simulink model "TrajectoryTracking_2015b_00"  (R2016a)
settings: Solver=ode45  SolverMode=SingleTasking  StartTime=0.0  StopTime=200  RelTol=1e-3
values from neighbouring files (symbols this model uses):
  B_input = B_T    [ErrorDynamicsControllerDesign.m]
undefined symbols (not defined in the file or in its folder): angular_velocity_pitch_1, angular_velocity_pitch_2, angular_velocity_pitch_3, angular_velocity_pitch_4, angular_velocity_pitch_5, angular_velocity_pitch_6, angular_velocity_roll_1, angular_velocity_roll_2, angular_velocity_roll_3, angular_velocity_roll_4, angular_velocity_roll_5, angular_velocity_roll_6, angular_velocity_roll_7, angular_velocity_yaw_1, angular_velocity_yaw_2, angular_velocity_yaw_3, angular_velocity_yaw_4, angular_velocity_yaw_5, angular_velocity_yaw_6, angular_velocity_yaw_7, K1, K2, K3, K4, K5, K6, K7, linear_velocity_x_1, linear_velocity_x_2, linear_velocity_x_3, linear_velocity_x_4, linear_velocity_x_5, linear_velocity_x_6, linear_velocity_x_7, linear_velocity_y_1, linear_velocity_y_2, linear_velocity_y_3, linear_velocity_y_4, linear_velocity_y_5, linear_velocity_y_6, linear_velocity_y_7, linear_velocity_z_1, linear_velocity_z_2, linear_velocity_z_3, linear_velocity_z_4, linear_velocity_z_5, linear_velocity_z_6, linear_velocity_z_7, pitch_angle_1, pitch_angle_2, pitch_angle_3, pitch_angle_4, pitch_angle_5, pitch_angle_6, pitch_angle_7, roll_angle_1, roll_angle_2, roll_angle_3, roll_angle_4, roll_angle_5 ... (+59)
undefined symbols (not defined in the file): b_T1_optimized, b_T2_optimized, b_T3_optimized, b_T4_optimized, b_T5_optimized, b_T6_optimized, d_T1_optimized, d_T2_optimized, d_T3_optimized, d_T4_optimized, d_T5_optimized, d_T6_optimized, r_T1_optimized, r_T2_optimized, r_T3_optimized, r_T4_optimized, r_T5_optimized, r_T6_optimized
libraries: aerolibtransform2 x1, aerolib6dofsys x1
(part 1 of 2)
settings Model: Creator=yongyu  LastModifiedBy=ychen
settings DebuggingCC: SFUnexpectedBacktrackingDiag=error  SFNoUnconditionalDefaultTransitionDiag=error
settings GRTTargetCC: TargetLangStandard=C99 (ISO)  GeneratePreprocessorConditionals=Use local settings
settings ConfigComp: CovMetricSettings=dwe  CovHtmlReporting=off  CovSaveCumulativeToWorkspaceVar=off  CovSaveSingleToWorkspaceVar=off  CovModelRefEnable=Off  CovExternalEMLEnable=on

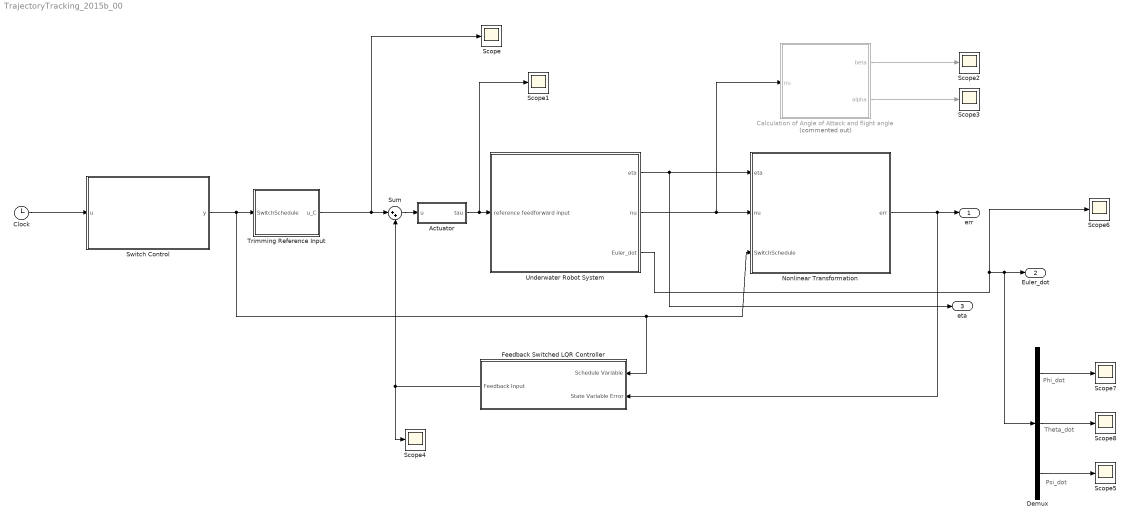
== system TrajectoryTracking_2015b_00 ==
  note: Theta_dot
  note: Phi_dot
  note: Psi_dot
  Actuator : Subsystem
  Calculation of Angle of Attack and flight angle : Subsystem  Commented=on
  Clock : Clock
  Demux : Demux  Outputs=3
  Feedback Switched LQR Controller : Subsystem
  Nonlinear Transformation : Subsystem
  Scope{,1..8} (9 alike) : Scope
  Sum : Sum  Inputs=|++
  Switch Control : MATLAB Function  TreatAsAtomicUnit=on
  "Trimming Reference Input " : Subsystem
  Underwater Robot System : Subsystem
  err : Outport
  Euler_dot : Outport  Port=2
  eta : Outport  Port=3
  wires:
  Nonlinear Transformation/1(err) -> err/1, Feedback Switched LQR Controller/2(State Variable Error)
  Calculation of Angle of Attack and flight angle/2(alpha) -> Scope3/1
  Calculation of Angle of Attack and flight angle/1(beta) -> Scope2/1
  "Trimming Reference Input "/1(u_C) -> Scope/1, Sum/1
  Underwater Robot System/1(eta) -> eta/1, Nonlinear Transformation/1(eta)
  Underwater Robot System/2(nu) -> Calculation of Angle of Attack and flight angle/1(nu), Nonlinear Transformation/2(nu)
  Underwater Robot System/3(Euler_dot) -> Scope6/1, Demux/1, Euler_dot/1
  Clock/1 -> Switch Control/1(u)
  Demux/3 -> Scope5/1
  Switch Control/1(y) -> Feedback Switched LQR Controller/1(Schedule Variable), Nonlinear Transformation/3(SwitchSchedule), "Trimming Reference Input "/1(SwitchSchedule)
  Demux/1 -> Scope7/1
  Demux/2 -> Scope8/1
  Sum/1 -> Actuator/1(u)
  Actuator/1(tau) -> Scope1/1, Underwater Robot System/1("reference feedforward input ")
  Feedback Switched LQR Controller/1(Feedback Input) -> Sum/2, Scope4/1

== system TrajectoryTracking_2015b_00/Actuator ==
  u : Inport
  Add : Sum  Inputs=++++++
  Demux : Demux  Outputs=6
  Saturation : Saturate  UpperLimit=[40 40 40 40 40 40]  LowerLimit=[-35 -35 -35 -35 -35 -35]
  Scope{1..6} (6 alike) : Scope
  Thruster Model1 : Subsystem  mask{d_T=d_T1_optimized, b_T=b_T1_optimized, r_T=r_T1_optimized, lambda_T=veh.lambda1}
      mask DialogControl DescTextVar Prompt: Model of Thruster
  Thruster Model2 : Subsystem  mask{d_T=d_T2_optimized, b_T=b_T2_optimized, r_T=r_T2_optimized, lambda_T=veh.lambda2}
      mask DialogControl DescTextVar Prompt: Model of Thruster
  Thruster Model3 : Subsystem  mask{d_T=d_T3_optimized, b_T=b_T3_optimized, r_T=r_T3_optimized, lambda_T=veh.lambda3}
      mask DialogControl DescTextVar Prompt: Model of Thruster
  Thruster Model4 : Subsystem  mask{d_T=d_T4_optimized, b_T=b_T4_optimized, r_T=r_T4_optimized, lambda_T=veh.lambda4}
      mask DialogControl DescTextVar Prompt: Model of Thruster
  Thruster Model5 : Subsystem  mask{d_T=d_T5_optimized, b_T=b_T5_optimized, r_T=r_T5_optimized, lambda_T=veh.lambda5}
      mask DialogControl DescTextVar Prompt: Model of Thruster
  Thruster Model6 : Subsystem  mask{d_T=d_T6_optimized, b_T=b_T6_optimized, r_T=r_T6_optimized, lambda_T=veh.lambda6}
      mask DialogControl DescTextVar Prompt: Model of Thruster
  tau : Outport
  wires:
  Thruster Model5/1(tau) -> Add/5
  Thruster Model3/1(tau) -> Add/3
  Thruster Model4/1(tau) -> Add/4
  Thruster Model2/1(tau) -> Add/2
  Thruster Model6/1(tau) -> Add/6
  Add/1 -> tau/1
  Thruster Model1/1(tau) -> Add/1
  Demux/1 -> Thruster Model1/1(u), Scope1/1
  Demux/2 -> Thruster Model2/1(u), Scope2/1
  Demux/3 -> Thruster Model3/1(u), Scope3/1
  Demux/4 -> Thruster Model4/1(u), Scope4/1
  Demux/5 -> Thruster Model5/1(u), Scope5/1
  Demux/6 -> Thruster Model6/1(u), Scope6/1
  u/1 -> Demux/1

== system TrajectoryTracking_2015b_00/Calculation of Angle of Attack and flight angle ==
  nu : Inport
  Add : Sum  Inputs=+++
  Add1 : Sum
  Demux : Demux  Outputs=3
  Demux1 : Demux  Outputs=2
  Divide : Product  Inputs=*/
  Divide1 : Product  Inputs=*/
  Product{,1..4} (5 alike) : Product
  Selector1 : Selector  InputPortWidth=6  IndexOptions=Index vector (dialog)  Indices=[1 2 3]  OutputSizes=1
  Selector2 : Selector  InputPortWidth=6  IndexOptions=Index vector (dialog)  Indices=[1 3]  OutputSizes=1
  Sqrt : Sqrt  SaturateOnIntegerOverflow=on
  Sqrt1 : Sqrt  SaturateOnIntegerOverflow=on
  beta : Outport
  alpha : Outport  Port=2
  wires:
  nu/1 -> Selector2/1, Selector1/1
  Selector1/1 -> Demux/1
  Demux/1 -> Product/2, Product/1
  Demux/2 -> Product1/2, Product1/1, Divide/1
  Demux/3 -> Product2/2, Product2/1
  Product/1 -> Add/1
  Product1/1 -> Add/2
  Product2/1 -> Add/3
  Add/1 -> Sqrt/1
  Sqrt/1 -> Divide/2
  Divide/1 -> beta/1
  Selector2/1 -> Demux1/1
  Demux1/1 -> Product3/2, Product3/1
  Demux1/2 -> Divide1/1, Product4/2, Product4/1
  Product3/1 -> Add1/1
  Product4/1 -> Add1/2
  Add1/1 -> Sqrt1/1
  Sqrt1/1 -> Divide1/2
  Divide1/1 -> alpha/1

== system TrajectoryTracking_2015b_00/Feedback Switched LQR Controller ==
  Schedule Variable : Inport
  State Variable Error : Inport  Port=2
  Constant1 : Constant  Value=-K2
  Constant2 : Constant  Value=-K3
  Constant3 : Constant  Value=-K4
  Constant4 : Constant  Value=-K5
  Constant5 : Constant  Value=-K6
  Constant6 : Constant  Value=-K7
  Constant7 : Constant  Value=-K1
  Multiport Switch : MultiPortSwitch  Inputs=7
  Product : Product  Multiplication=Matrix(*)
  Feedback Input : Outport
  wires:
  Constant7/1 -> Multiport Switch/2
  Constant1/1 -> Multiport Switch/3
  Constant2/1 -> Multiport Switch/4
  Constant3/1 -> Multiport Switch/5
  Multiport Switch/1 -> Product/1
  Constant4/1 -> Multiport Switch/6
  Constant5/1 -> Multiport Switch/7
  Constant6/1 -> Multiport Switch/8
  Product/1 -> Feedback Input/1
  State Variable Error/1 -> Product/2
  Schedule Variable/1 -> Multiport Switch/1

== system TrajectoryTracking_2015b_00/Nonlinear Transformation ==
  eta : Inport
  nu : Inport  Port=2
  SwitchSchedule : Inport  Port=3
  Mux2 : Mux
  "Position Error " : Subsystem
  Scope{,1..3} (4 alike) : Scope
  Transfer Fcn : TransferFcn
  "Velocity Error " : Subsystem
  surge,sway,yaw,roll,pitch,yaw : Scope
  x,y,z,phi,theta,psi : Scope
  err : Outport
  wires:
  nu/1 -> surge,sway,yaw,roll,pitch,yaw/1, "Velocity Error "/1(vel)
  eta/1 -> x,y,z,phi,theta,psi/1, "Position Error "/1(pos)
  Mux2/1 -> err/1
  "Position Error "/1(p_E) -> Scope/1, Mux2/1
  "Position Error "/2(lambda_E) -> Scope1/1, Mux2/2
  "Velocity Error "/1(nu_err) -> Scope3/1, Mux2/3
  "Velocity Error "/2(omega_err) -> Scope2/1, Mux2/4
  SwitchSchedule/1 -> "Position Error "/2(SwitchSchedule), "Velocity Error "/2(SwitchSchedule)

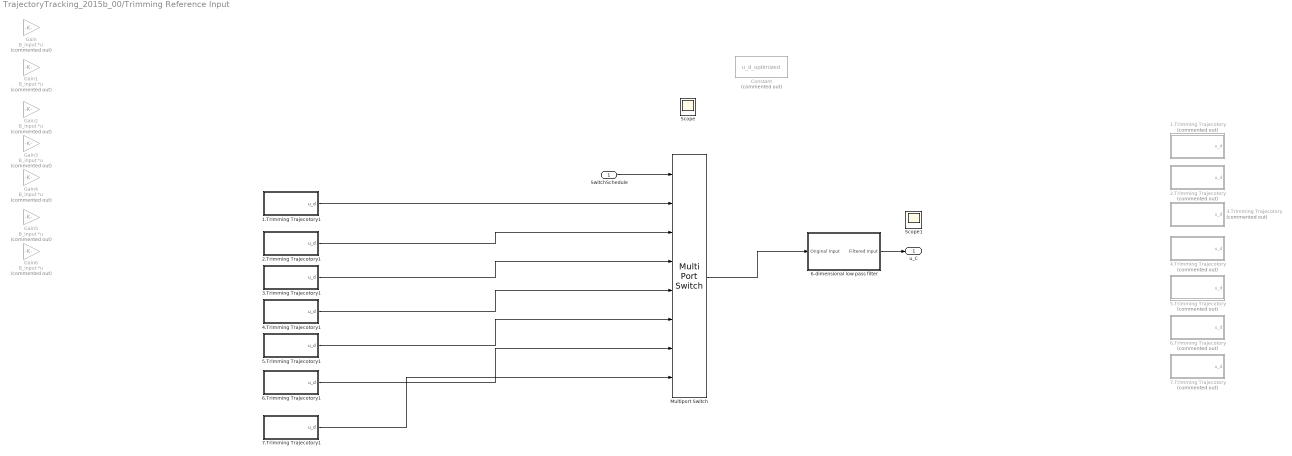
== system TrajectoryTracking_2015b_00/Trimming Reference Input  ==
  SwitchSchedule : Inport
  1.Trimming Trajecotory : Subsystem  Commented=on
  1.Trimming Trajecotory1 : Subsystem
  2.Trimming Trajecotory : Subsystem  Commented=on
  2.Trimming Trajecotory1 : Subsystem
  3.Trimming Trajecotory : Subsystem  Commented=on
  3.Trimming Trajecotory1 : Subsystem
  4.Trimming Trajecotory : Subsystem  Commented=on
  4.Trimming Trajecotory1 : Subsystem
  5.Trimming Trajecotory : Subsystem  Commented=on
  5.Trimming Trajecotory1 : Subsystem
  6-dimensional low pass filter : Subsystem
  6.Trimming Trajecotory : Subsystem  Commented=on
  6.Trimming Trajecotory1 : Subsystem
  7.Trimming Trajecotory : Subsystem  Commented=on
  7.Trimming Trajecotory1 : Subsystem
  Constant : Constant  Commented=on  Value=u_d_optimized
  Gain{,1..6} (7 alike) : Gain  Commented=on  Gain=B_input  Multiplication=Matrix(K*u)
  Multiport Switch : MultiPortSwitch  Inputs=7
  Scope : Scope
  Scope1 : Scope
  u_C : Outport
  wires:
  SwitchSchedule/1 -> Multiport Switch/1
  2.Trimming Trajecotory1/1(u_d) -> Multiport Switch/3
  3.Trimming Trajecotory1/1(u_d) -> Multiport Switch/4
  4.Trimming Trajecotory1/1(u_d) -> Multiport Switch/5
  5.Trimming Trajecotory1/1(u_d) -> Multiport Switch/6
  6.Trimming Trajecotory1/1(u_d) -> Multiport Switch/7
  7.Trimming Trajecotory1/1(u_d) -> Multiport Switch/8
  1.Trimming Trajecotory1/1(u_d) -> Multiport Switch/2
  6-dimensional low pass filter/1(Filtered Input) -> u_C/1
  Multiport Switch/1 -> 6-dimensional low pass filter/1(Original Input)

== system TrajectoryTracking_2015b_00/Underwater Robot System ==
  "reference feedforward input " : Inport
  Demux : Demux  Outputs=6
  Underwater Robot System : Subsystem
  eta : Outport
  nu : Outport  Port=2
  Euler_dot : Outport  Port=3
  wires:
  Underwater Robot System/1(eta) -> eta/1
  Underwater Robot System/2(nu) -> nu/1
  Demux/6 -> Underwater Robot System/6(N)
  Demux/5 -> Underwater Robot System/5(M)
  Demux/4 -> Underwater Robot System/4(K)
  Demux/3 -> Underwater Robot System/3(Z)
  Demux/2 -> Underwater Robot System/2(Y)
  Demux/1 -> Underwater Robot System/1(X)
  "reference feedforward input "/1 -> Demux/1
  Underwater Robot System/3(Euler_dot) -> Euler_dot/1

== system TrajectoryTracking_2015b_00/Actuator/Thruster Model1 ==
  u : Inport
  3x3 cross product : Subsystem
  Constant : Constant  Value=r_T
  Constant1 : Constant  Value=d_T
  Display : Display
  Gain : Gain  Gain=d_T  Multiplication=Matrix(K*u)
  Gain1 : Gain  Gain=b_T*lambda_T*d_T  Multiplication=Matrix(K*u)
  Mux : Mux  Inputs=2
  Product : Product
  Sum : Sum  Inputs=|++
  tau : Outport
  wires:
  u/1 -> Product/1, Gain1/1, Gain/1
  Constant/1 -> 3x3 cross product/1(a)
  Constant1/1 -> 3x3 cross product/2(b)
  Gain1/1 -> Sum/1
  3x3 cross product/1(c) -> Product/2
  Gain/1 -> Mux/1
  Mux/1 -> tau/1
  Sum/1 -> Mux/2
  Product/1 -> Sum/2, Display/1

== system TrajectoryTracking_2015b_00/Actuator/Thruster Model2 ==
  u : Inport
  3x3 cross product : Subsystem
  Constant : Constant  Value=r_T
  Constant1 : Constant  Value=d_T
  Display : Display
  Gain : Gain  Gain=d_T  Multiplication=Matrix(K*u)
  Gain1 : Gain  Gain=b_T*lambda_T*d_T  Multiplication=Matrix(K*u)
  Mux : Mux  Inputs=2
  Product : Product
  Sum : Sum  Inputs=|++
  tau : Outport
  wires:
  u/1 -> Product/1, Gain1/1, Gain/1
  Constant/1 -> 3x3 cross product/1(a)
  Constant1/1 -> 3x3 cross product/2(b)
  Gain1/1 -> Sum/1
  3x3 cross product/1(c) -> Product/2
  Gain/1 -> Mux/1
  Mux/1 -> tau/1
  Sum/1 -> Mux/2
  Product/1 -> Sum/2, Display/1

== system TrajectoryTracking_2015b_00/Actuator/Thruster Model3 ==
  u : Inport
  3x3 cross product : Subsystem
  Constant : Constant  Value=r_T
  Constant1 : Constant  Value=d_T
  Display : Display
  Gain : Gain  Gain=d_T  Multiplication=Matrix(K*u)
  Gain1 : Gain  Gain=b_T*lambda_T*d_T  Multiplication=Matrix(K*u)
  Mux : Mux  Inputs=2
  Product : Product
  Sum : Sum  Inputs=|++
  tau : Outport
  wires:
  u/1 -> Product/1, Gain1/1, Gain/1
  Constant/1 -> 3x3 cross product/1(a)
  Constant1/1 -> 3x3 cross product/2(b)
  Gain1/1 -> Sum/1
  3x3 cross product/1(c) -> Product/2
  Gain/1 -> Mux/1
  Mux/1 -> tau/1
  Sum/1 -> Mux/2
  Product/1 -> Sum/2, Display/1

== system TrajectoryTracking_2015b_00/Actuator/Thruster Model4 ==
  u : Inport
  3x3 cross product : Subsystem
  Constant : Constant  Value=r_T
  Constant1 : Constant  Value=d_T
  Display : Display
  Gain : Gain  Gain=d_T  Multiplication=Matrix(K*u)
  Gain1 : Gain  Gain=b_T*lambda_T*d_T  Multiplication=Matrix(K*u)
  Mux : Mux  Inputs=2
  Product : Product
  Sum : Sum  Inputs=|++
  tau : Outport
  wires:
  u/1 -> Product/1, Gain1/1, Gain/1
  Constant/1 -> 3x3 cross product/1(a)
  Constant1/1 -> 3x3 cross product/2(b)
  Gain1/1 -> Sum/1
  3x3 cross product/1(c) -> Product/2
  Gain/1 -> Mux/1
  Mux/1 -> tau/1
  Sum/1 -> Mux/2
  Product/1 -> Sum/2, Display/1

== system TrajectoryTracking_2015b_00/Actuator/Thruster Model5 ==
  u : Inport
  3x3 cross product : Subsystem
  Constant : Constant  Value=r_T
  Constant1 : Constant  Value=d_T
  Display : Display
  Gain : Gain  Gain=d_T  Multiplication=Matrix(K*u)
  Gain1 : Gain  Gain=b_T*lambda_T*d_T  Multiplication=Matrix(K*u)
  Mux : Mux  Inputs=2
  Product : Product
  Sum : Sum  Inputs=|++
  tau : Outport
  wires:
  u/1 -> Product/1, Gain1/1, Gain/1
  Constant/1 -> 3x3 cross product/1(a)
  Constant1/1 -> 3x3 cross product/2(b)
  Gain1/1 -> Sum/1
  3x3 cross product/1(c) -> Product/2
  Gain/1 -> Mux/1
  Mux/1 -> tau/1
  Sum/1 -> Mux/2
  Product/1 -> Sum/2, Display/1

== system TrajectoryTracking_2015b_00/Actuator/Thruster Model6 ==
  u : Inport
  3x3 cross product : Subsystem
  Constant : Constant  Value=r_T
  Constant1 : Constant  Value=d_T
  Display : Display
  Gain : Gain  Gain=d_T  Multiplication=Matrix(K*u)
  Gain1 : Gain  Gain=b_T*lambda_T*d_T  Multiplication=Matrix(K*u)
  Mux : Mux  Inputs=2
  Product : Product
  Sum : Sum  Inputs=|++
  tau : Outport
  wires:
  u/1 -> Product/1, Gain1/1, Gain/1
  Constant/1 -> 3x3 cross product/1(a)
  Constant1/1 -> 3x3 cross product/2(b)
  Gain1/1 -> Sum/1
  3x3 cross product/1(c) -> Product/2
  Gain/1 -> Mux/1
  Mux/1 -> tau/1
  Sum/1 -> Mux/2
  Product/1 -> Sum/2, Display/1

== system TrajectoryTracking_2015b_00/Nonlinear Transformation/Position Error  ==
  pos : Inport
  SwitchSchedule : Inport  Port=2
  Nonlinear Orientation Transformation : Subsystem
  Nonlinear Position Transformation : Subsystem
  Selector1 : Selector  InputPortWidth=6  IndexOptions=Index vector (dialog)  Indices=[1 2 3]  OutputSizes=1
  Selector2 : Selector  InputPortWidth=6  IndexOptions=Index vector (dialog)  Indices=[4 5 6]  OutputSizes=1
  p_E : Outport
  lambda_E : Outport  Port=2
  wires:
  pos/1 -> Selector2/1, Selector1/1
  Selector2/1 -> Nonlinear Position Transformation/2(theta), Nonlinear Orientation Transformation/1(theta)
  Selector1/1 -> Nonlinear Position Transformation/1(x,y,z)
  Nonlinear Position Transformation/1(p_E) -> p_E/1
  Nonlinear Orientation Transformation/1(lambda_E) -> lambda_E/1
  SwitchSchedule/1 -> Nonlinear Orientation Transformation/2(SwitchSchedule), Nonlinear Position Transformation/3(SwitchSchedule)

== system TrajectoryTracking_2015b_00/Nonlinear Transformation/Velocity Error  ==
  vel : Inport
  SwitchSchedule : Inport  Port=2
  Demux : Demux  Outputs=6
  Mux : Mux  Inputs=3
  Mux1 : Mux  Inputs=3
  heave_error : Subsystem
  pitch_error : Subsystem
  roll_error : Subsystem
  surge_error : Subsystem
  sway_error : Subsystem
  yaw_error : Subsystem
  nu_err : Outport
  omega_err : Outport  Port=2
  wires:
  vel/1 -> Demux/1
  Mux/1 -> nu_err/1
  Demux/1 -> surge_error/1(surge)
  Demux/2 -> sway_error/1(sway)
  Demux/3 -> heave_error/1(heave)
  Demux/4 -> roll_error/1(roll)
  Demux/5 -> pitch_error/1(pitch)
  Demux/6 -> yaw_error/1(pitch)
  surge_error/1(surge_err) -> Mux/1
  sway_error/1(sway_err) -> Mux/2
  heave_error/1(heave_err) -> Mux/3
  roll_error/1(roll_err) -> Mux1/1
  pitch_error/1(pitch_err) -> Mux1/2
  yaw_error/1(pitch_err) -> Mux1/3
  Mux1/1 -> omega_err/1
  SwitchSchedule/1 -> yaw_error/2(SwitchSchedule), pitch_error/2(SwitchSchedule), roll_error/2(SwitchSchedule), sway_error/2(SwitchSchedule), surge_error/2(SwitchSchedule), heave_error/2(SwitchSchedule)

== system TrajectoryTracking_2015b_00/Trimming Reference Input /1.Trimming Trajecotory ==
  Constant : Constant  Value=tau_d_1(1,1,1)
  Constant1 : Constant  Value=tau_d_1(2,1,1)
  Constant2 : Constant  Value=tau_d_1(3,1,1)
  Constant3 : Constant  Value=tau_d_1(4,1,1)
  Constant4 : Constant  Value=tau_d_1(5,1,1)
  Constant5 : Constant  Value=tau_d_1(6,1,1)
  Mux : Mux  Inputs=6
  u_d : Outport
  wires:
  Mux/1 -> u_d/1
  Constant/1 -> Mux/1
  Constant1/1 -> Mux/2
  Constant2/1 -> Mux/3
  Constant3/1 -> Mux/4
  Constant4/1 -> Mux/5
  Constant5/1 -> Mux/6

== system TrajectoryTracking_2015b_00/Trimming Reference Input /1.Trimming Trajecotory1 ==
  Constant : Constant  Value=u_d_1
  u_d : Outport
  wires:
  Constant/1 -> u_d/1

== system TrajectoryTracking_2015b_00/Trimming Reference Input /2.Trimming Trajecotory ==
  Constant : Constant  Value=tau_d_2(1,1,1)
  Constant1 : Constant  Value=tau_d_2(2,1,1)
  Constant2 : Constant  Value=tau_d_2(3,1,1)
  Constant3 : Constant  Value=tau_d_2(4,1,1)
  Constant4 : Constant  Value=tau_d_2(5,1,1)
  Constant5 : Constant  Value=tau_d_2(6,1,1)
  Mux : Mux  Inputs=6
  u_d : Outport
  wires:
  Constant4/1 -> Mux/5
  Constant3/1 -> Mux/4
  Constant5/1 -> Mux/6
  Constant2/1 -> Mux/3
  Constant/1 -> Mux/1
  Mux/1 -> u_d/1
  Constant1/1 -> Mux/2

== system TrajectoryTracking_2015b_00/Trimming Reference Input /2.Trimming Trajecotory1 ==
  Constant : Constant  Value=u_d_2
  u_d : Outport
  wires:
  Constant/1 -> u_d/1

== system TrajectoryTracking_2015b_00/Trimming Reference Input /3.Trimming Trajecotory ==
  Constant : Constant  Value=tau_d_3(1,1,1)
  Constant1 : Constant  Value=tau_d_3(2,1,1)
  Constant2 : Constant  Value=tau_d_3(3,1,1)
  Constant3 : Constant  Value=tau_d_3(4,1,1)
  Constant4 : Constant  Value=tau_d_3(5,1,1)
  Constant5 : Constant  Value=tau_d_3(6,1,1)
  Mux : Mux  Inputs=6
  u_d : Outport
  wires:
  Constant3/1 -> Mux/4
  Mux/1 -> u_d/1
  Constant5/1 -> Mux/6
  Constant2/1 -> Mux/3
  Constant4/1 -> Mux/5
  Constant/1 -> Mux/1
  Constant1/1 -> Mux/2

== system TrajectoryTracking_2015b_00/Trimming Reference Input /3.Trimming Trajecotory1 ==
  Constant : Constant  Value=u_d_3
  u_d : Outport
  wires:
  Constant/1 -> u_d/1

== system TrajectoryTracking_2015b_00/Trimming Reference Input /4.Trimming Trajecotory ==
  Constant : Constant  Value=tau_d_4(1,1,1)
  Constant1 : Constant  Value=tau_d_4(2,1,1)
  Constant2 : Constant  Value=tau_d_4(3,1,1)
  Constant3 : Constant  Value=tau_d_4(4,1,1)
  Constant4 : Constant  Value=tau_d_4(5,1,1)
  Constant5 : Constant  Value=tau_d_4(6,1,1)
  Mux : Mux  Inputs=6
  u_d : Outport
  wires:
  Constant1/1 -> Mux/2
  Constant/1 -> Mux/1
  Constant4/1 -> Mux/5
  Constant2/1 -> Mux/3
  Constant5/1 -> Mux/6
  Mux/1 -> u_d/1
  Constant3/1 -> Mux/4

== system TrajectoryTracking_2015b_00/Trimming Reference Input /4.Trimming Trajecotory1 ==
  Constant : Constant  Value=u_d_4
  u_d : Outport
  wires:
  Constant/1 -> u_d/1

== system TrajectoryTracking_2015b_00/Trimming Reference Input /5.Trimming Trajecotory ==
  Constant : Constant  Value=tau_d_5(1,1,1)
  Constant1 : Constant  Value=tau_d_5(2,1,1)
  Constant2 : Constant  Value=tau_d_5(3,1,1)
  Constant3 : Constant  Value=tau_d_5(4,1,1)
  Constant4 : Constant  Value=tau_d_5(5,1,1)
  Constant5 : Constant  Value=tau_d_5(6,1,1)
  Mux : Mux  Inputs=6
  u_d : Outport
  wires:
  Constant1/1 -> Mux/2
  Constant/1 -> Mux/1
  Constant4/1 -> Mux/5
  Constant2/1 -> Mux/3
  Constant5/1 -> Mux/6
  Mux/1 -> u_d/1
  Constant3/1 -> Mux/4

== system TrajectoryTracking_2015b_00/Trimming Reference Input /5.Trimming Trajecotory1 ==
  Constant : Constant  Value=u_d_5
  u_d : Outport
  wires:
  Constant/1 -> u_d/1

== system TrajectoryTracking_2015b_00/Trimming Reference Input /6-dimensional low pass filter ==
  Original Input : Inport
  Demux : Demux  Outputs=6
  Mux : Mux  Inputs=6
  Transfer Fcn{,1..5} (6 alike) : TransferFcn  Denominator=[1 1]
  Filtered Input : Outport
  wires:
  Transfer Fcn/1 -> Mux/1
  Demux/5 -> Transfer Fcn4/1
  Demux/2 -> Transfer Fcn1/1
  Transfer Fcn3/1 -> Mux/4
  Demux/4 -> Transfer Fcn3/1
  Demux/3 -> Transfer Fcn2/1
  Transfer Fcn4/1 -> Mux/5
  Transfer Fcn5/1 -> Mux/6
  Demux/1 -> Transfer Fcn/1
  Transfer Fcn1/1 -> Mux/2
  Transfer Fcn2/1 -> Mux/3
  Demux/6 -> Transfer Fcn5/1
  Mux/1 -> Filtered Input/1
  Original Input/1 -> Demux/1

== system TrajectoryTracking_2015b_00/Trimming Reference Input /6.Trimming Trajecotory ==
  Constant : Constant  Value=tau_d_6(1,1,1)
  Constant1 : Constant  Value=tau_d_6(2,1,1)
  Constant2 : Constant  Value=tau_d_6(3,1,1)
  Constant3 : Constant  Value=tau_d_6(4,1,1)
  Constant4 : Constant  Value=tau_d_6(5,1,1)
  Constant5 : Constant  Value=tau_d_6(6,1,1)
  Mux : Mux  Inputs=6
  u_d : Outport
  wires:
  Constant1/1 -> Mux/2
  Constant/1 -> Mux/1
  Constant4/1 -> Mux/5
  Constant2/1 -> Mux/3
  Constant5/1 -> Mux/6
  Mux/1 -> u_d/1
  Constant3/1 -> Mux/4

== system TrajectoryTracking_2015b_00/Trimming Reference Input /6.Trimming Trajecotory1 ==
  Constant : Constant  Value=u_d_6
  u_d : Outport
  wires:
  Constant/1 -> u_d/1

== system TrajectoryTracking_2015b_00/Trimming Reference Input /7.Trimming Trajecotory ==
  Constant : Constant  Value=tau_d_7(1,1,1)
  Constant1 : Constant  Value=tau_d_7(2,1,1)
  Constant2 : Constant  Value=tau_d_7(3,1,1)
  Constant3 : Constant  Value=tau_d_7(4,1,1)
  Constant4 : Constant  Value=tau_d_7(5,1,1)
  Constant5 : Constant  Value=tau_d_7(6,1,1)
  Mux : Mux  Inputs=6
  u_d : Outport
  wires:
  Constant1/1 -> Mux/2
  Constant/1 -> Mux/1
  Constant4/1 -> Mux/5
  Constant2/1 -> Mux/3
  Constant5/1 -> Mux/6
  Mux/1 -> u_d/1
  Constant3/1 -> Mux/4

== system TrajectoryTracking_2015b_00/Trimming Reference Input /7.Trimming Trajecotory1 ==
  Constant : Constant  Value=u_d_7
  u_d : Outport
  wires:
  Constant/1 -> u_d/1

== system TrajectoryTracking_2015b_00/Underwater Robot System/Underwater Robot System ==
  X : Inport
  Y : Inport  Port=2
  Z : Inport  Port=3
  K : Inport  Port=4
  M : Inport  Port=5
  N : Inport  Port=6
  Display : Display
  Display1 : Display
  DragCalculation : Subsystem
  Dynamic2Kinematic(angular velocity) : Subsystem
  Initial Integration Value Generation Generalised Location : Subsystem
  Mux : Mux  Inputs=2
  Mux1 : Mux  Inputs=2
  Mux2 : Mux  Inputs=6
  Position Integrator(x,y,z) : Integrator  InitialConditionSource=external
  Scope : Scope
  Sum : Sum  Inputs=|+-
  Transpose : Math  Operator=transpose  SaturateOnIntegerOverflow=on
  "Underwater Robot Dynamics " : Subsystem
  "transform to inertial world frame {i}" : Subsystem
  eta : Outport
  nu : Outport  Port=2
  Euler_dot : Outport  Port=3
  wires:
  Transpose/1 -> "transform to inertial world frame {i}"/2(linear velocity transformation matrix)
  Mux1/1 -> nu/1, DragCalculation/1(nu)  "nu"
  Mux/1 -> eta/1
  "transform to inertial world frame {i}"/1(Ve) -> Position Integrator(x,y,z)/1
  Position Integrator(x,y,z)/1 -> Mux/1
  "Underwater Robot Dynamics "/2(w_ib) -> Mux1/2, Dynamic2Kinematic(angular velocity)/1("p q r ")
  "Underwater Robot Dynamics "/1(v) -> Mux1/1, "transform to inertial world frame {i}"/1(v)
  N/1 -> Mux2/6
  M/1 -> Mux2/5
  K/1 -> Mux2/4
  Z/1 -> Mux2/3
  Y/1 -> Mux2/2
  X/1 -> Mux2/1
  Dynamic2Kinematic(angular velocity)/1(DCM) -> Transpose/1
  Dynamic2Kinematic(angular velocity)/2(Euler) -> Mux/2
  Initial Integration Value Generation Generalised Location/1(Initial Location Integration Value) -> Position Integrator(x,y,z)/2
  Dynamic2Kinematic(angular velocity)/3(Euler_dot) -> Euler_dot/1
  DragCalculation/1(HullDrag) -> Scope/1, Display1/1, Sum/2
  Mux2/1 -> Sum/1
  Sum/1 -> "Underwater Robot Dynamics "/1(tau_b)

== system TrajectoryTracking_2015b_00/Actuator/Thruster Model1/3x3 cross product ==
  a : Inport
  b : Inport  Port=2
  Product : Product  SaturateOnIntegerOverflow=on  InputSameDT=on  OutDataTypeStr=Inherit: Same as first input
  Product1 : Product  SaturateOnIntegerOverflow=on  InputSameDT=on  OutDataTypeStr=Inherit: Same as first input
  Selector : Selector  InputPortWidth=3  IndexOptions=Index vector (dialog)  Indices=[2 3 1]  OutputSizes=1
  Selector1 : Selector  InputPortWidth=3  IndexOptions=Index vector (dialog)  Indices=[3 1 2]  OutputSizes=1
  Selector2 : Selector  InputPortWidth=3  IndexOptions=Index vector (dialog)  Indices=[2 3 1]  OutputSizes=1
  Selector3 : Selector  InputPortWidth=3  IndexOptions=Index vector (dialog)  Indices=[3 1 2]  OutputSizes=1
  Sum : Sum  Inputs=+|-  SaturateOnIntegerOverflow=on  InputSameDT=on  OutDataTypeStr=Inherit: Same as first input
  c : Outport  InitialOutput=0
  wires:
  Selector3/1 -> Product1/1
  Selector2/1 -> Product1/2
  Product1/1 -> Sum/2
  Selector1/1 -> Product/2
  Product/1 -> Sum/1
  a/1 -> Selector3/1, Selector/1
  Selector/1 -> Product/1
  b/1 -> Selector2/1, Selector1/1
  Sum/1 -> c/1

== system TrajectoryTracking_2015b_00/Actuator/Thruster Model2/3x3 cross product ==
  a : Inport
  b : Inport  Port=2
  Product : Product  SaturateOnIntegerOverflow=on  InputSameDT=on  OutDataTypeStr=Inherit: Same as first input
  Product1 : Product  SaturateOnIntegerOverflow=on  InputSameDT=on  OutDataTypeStr=Inherit: Same as first input
  Selector : Selector  InputPortWidth=3  IndexOptions=Index vector (dialog)  Indices=[2 3 1]  OutputSizes=1
  Selector1 : Selector  InputPortWidth=3  IndexOptions=Index vector (dialog)  Indices=[3 1 2]  OutputSizes=1
  Selector2 : Selector  InputPortWidth=3  IndexOptions=Index vector (dialog)  Indices=[2 3 1]  OutputSizes=1
  Selector3 : Selector  InputPortWidth=3  IndexOptions=Index vector (dialog)  Indices=[3 1 2]  OutputSizes=1
  Sum : Sum  Inputs=+|-  SaturateOnIntegerOverflow=on  InputSameDT=on  OutDataTypeStr=Inherit: Same as first input
  c : Outport  InitialOutput=0
  wires:
  Selector3/1 -> Product1/1
  Selector2/1 -> Product1/2
  Product1/1 -> Sum/2
  Selector1/1 -> Product/2
  Product/1 -> Sum/1
  a/1 -> Selector3/1, Selector/1
  Selector/1 -> Product/1
  b/1 -> Selector2/1, Selector1/1
  Sum/1 -> c/1

== system TrajectoryTracking_2015b_00/Actuator/Thruster Model3/3x3 cross product ==
  a : Inport
  b : Inport  Port=2
  Product : Product  SaturateOnIntegerOverflow=on  InputSameDT=on  OutDataTypeStr=Inherit: Same as first input
  Product1 : Product  SaturateOnIntegerOverflow=on  InputSameDT=on  OutDataTypeStr=Inherit: Same as first input
  Selector : Selector  InputPortWidth=3  IndexOptions=Index vector (dialog)  Indices=[2 3 1]  OutputSizes=1
  Selector1 : Selector  InputPortWidth=3  IndexOptions=Index vector (dialog)  Indices=[3 1 2]  OutputSizes=1
  Selector2 : Selector  InputPortWidth=3  IndexOptions=Index vector (dialog)  Indices=[2 3 1]  OutputSizes=1
  Selector3 : Selector  InputPortWidth=3  IndexOptions=Index vector (dialog)  Indices=[3 1 2]  OutputSizes=1
  Sum : Sum  Inputs=+|-  SaturateOnIntegerOverflow=on  InputSameDT=on  OutDataTypeStr=Inherit: Same as first input
  c : Outport  InitialOutput=0
  wires:
  Selector3/1 -> Product1/1
  Selector2/1 -> Product1/2
  Product1/1 -> Sum/2
  Selector1/1 -> Product/2
  Product/1 -> Sum/1
  a/1 -> Selector3/1, Selector/1
  Selector/1 -> Product/1
  b/1 -> Selector2/1, Selector1/1
  Sum/1 -> c/1

== system TrajectoryTracking_2015b_00/Actuator/Thruster Model4/3x3 cross product ==
  a : Inport
  b : Inport  Port=2
  Product : Product  SaturateOnIntegerOverflow=on  InputSameDT=on  OutDataTypeStr=Inherit: Same as first input
  Product1 : Product  SaturateOnIntegerOverflow=on  InputSameDT=on  OutDataTypeStr=Inherit: Same as first input
  Selector : Selector  InputPortWidth=3  IndexOptions=Index vector (dialog)  Indices=[2 3 1]  OutputSizes=1
  Selector1 : Selector  InputPortWidth=3  IndexOptions=Index vector (dialog)  Indices=[3 1 2]  OutputSizes=1
  Selector2 : Selector  InputPortWidth=3  IndexOptions=Index vector (dialog)  Indices=[2 3 1]  OutputSizes=1
  Selector3 : Selector  InputPortWidth=3  IndexOptions=Index vector (dialog)  Indices=[3 1 2]  OutputSizes=1
  Sum : Sum  Inputs=+|-  SaturateOnIntegerOverflow=on  InputSameDT=on  OutDataTypeStr=Inherit: Same as first input
  c : Outport  InitialOutput=0
  wires:
  Selector3/1 -> Product1/1
  Selector2/1 -> Product1/2
  Product1/1 -> Sum/2
  Selector1/1 -> Product/2
  Product/1 -> Sum/1
  a/1 -> Selector3/1, Selector/1
  Selector/1 -> Product/1
  b/1 -> Selector2/1, Selector1/1
  Sum/1 -> c/1

== system TrajectoryTracking_2015b_00/Actuator/Thruster Model5/3x3 cross product ==
  a : Inport
  b : Inport  Port=2
  Product : Product  SaturateOnIntegerOverflow=on  InputSameDT=on  OutDataTypeStr=Inherit: Same as first input
  Product1 : Product  SaturateOnIntegerOverflow=on  InputSameDT=on  OutDataTypeStr=Inherit: Same as first input
  Selector : Selector  InputPortWidth=3  IndexOptions=Index vector (dialog)  Indices=[2 3 1]  OutputSizes=1
  Selector1 : Selector  InputPortWidth=3  IndexOptions=Index vector (dialog)  Indices=[3 1 2]  OutputSizes=1
  Selector2 : Selector  InputPortWidth=3  IndexOptions=Index vector (dialog)  Indices=[2 3 1]  OutputSizes=1
  Selector3 : Selector  InputPortWidth=3  IndexOptions=Index vector (dialog)  Indices=[3 1 2]  OutputSizes=1
  Sum : Sum  Inputs=+|-  SaturateOnIntegerOverflow=on  InputSameDT=on  OutDataTypeStr=Inherit: Same as first input
  c : Outport  InitialOutput=0
  wires:
  Selector3/1 -> Product1/1
  Selector2/1 -> Product1/2
  Product1/1 -> Sum/2
  Selector1/1 -> Product/2
  Product/1 -> Sum/1
  a/1 -> Selector3/1, Selector/1
  Selector/1 -> Product/1
  b/1 -> Selector2/1, Selector1/1
  Sum/1 -> c/1

== system TrajectoryTracking_2015b_00/Actuator/Thruster Model6/3x3 cross product ==
  a : Inport
  b : Inport  Port=2
  Product : Product  SaturateOnIntegerOverflow=on  InputSameDT=on  OutDataTypeStr=Inherit: Same as first input
  Product1 : Product  SaturateOnIntegerOverflow=on  InputSameDT=on  OutDataTypeStr=Inherit: Same as first input
  Selector : Selector  InputPortWidth=3  IndexOptions=Index vector (dialog)  Indices=[2 3 1]  OutputSizes=1
  Selector1 : Selector  InputPortWidth=3  IndexOptions=Index vector (dialog)  Indices=[3 1 2]  OutputSizes=1
  Selector2 : Selector  InputPortWidth=3  IndexOptions=Index vector (dialog)  Indices=[2 3 1]  OutputSizes=1
  Selector3 : Selector  InputPortWidth=3  IndexOptions=Index vector (dialog)  Indices=[3 1 2]  OutputSizes=1
  Sum : Sum  Inputs=+|-  SaturateOnIntegerOverflow=on  InputSameDT=on  OutDataTypeStr=Inherit: Same as first input
  c : Outport  InitialOutput=0
  wires:
  Selector3/1 -> Product1/1
  Selector2/1 -> Product1/2
  Product1/1 -> Sum/2
  Selector1/1 -> Product/2
  Product/1 -> Sum/1
  a/1 -> Selector3/1, Selector/1
  Selector/1 -> Product/1
  b/1 -> Selector2/1, Selector1/1
  Sum/1 -> c/1

== system TrajectoryTracking_2015b_00/Nonlinear Transformation/Position Error /Nonlinear Orientation Transformation ==
  theta : Inport
  SwitchSchedule : Inport  Port=2
  Demux : Demux  Outputs=3
  Display : Display
  Euler Angles to Angular Velocity Transfomration matrix : Subsystem
  Mux : Mux  Inputs=3
  Product : Product  Multiplication=Matrix(*)
  Transpose : Math  Operator=transpose  SaturateOnIntegerOverflow=on
  pitch_error : Subsystem
  roll_error : Subsystem
  yaw_error : Subsystem
  lambda_E : Outport
  wires:
  roll_error/1(roll_err) -> Mux/1
  yaw_error/1(yaw_err) -> Mux/3
  Demux/2 -> pitch_error/1(pitch)
  pitch_error/1(pitch_err) -> Mux/2
  Demux/3 -> yaw_error/1(yaw)
  theta/1 -> Euler Angles to Angular Velocity Transfomration matrix/1(theta), Demux/1
  Demux/1 -> roll_error/1(roll)
  Euler Angles to Angular Velocity Transfomration matrix/1(T) -> Transpose/1
  Transpose/1 -> Display/1, Product/1
  Mux/1 -> Product/2
  Product/1 -> lambda_E/1
  SwitchSchedule/1 -> yaw_error/2(SwitchSchedule), pitch_error/2(SwitchSchedule), roll_error/2(SwitchSchedule)

== system TrajectoryTracking_2015b_00/Nonlinear Transformation/Position Error /Nonlinear Position Transformation ==
  x,y,z : Inport
  theta : Inport  Port=2
  SwitchSchedule : Inport  Port=3
  Demux : Demux  Outputs=3
  Display : Display
  Euler Angles to inverse rotation matrix : Subsystem
  Mux : Mux  Inputs=3
  Product : Product  Multiplication=Matrix(*)
  x_error : Subsystem
  y_error : Subsystem
  z_error : Subsystem
  p_E : Outport
  wires:
  theta/1 -> Euler Angles to inverse rotation matrix/1(theta)
  Demux/3 -> z_error/1(z)
  Demux/2 -> y_error/1(y)
  Demux/1 -> x_error/1(x)
  x,y,z/1 -> Demux/1
  Product/1 -> p_E/1
  Mux/1 -> Product/2
  z_error/1(z_err) -> Mux/3
  x_error/1(x_err) -> Mux/1
  y_error/1(y_err) -> Mux/2
  Euler Angles to inverse rotation matrix/1(inv(R)) -> Display/1, Product/1
  SwitchSchedule/1 -> z_error/2(SwitchSchedule), y_error/2(SwitchSchedule), x_error/2(SwitchSchedule)

== system TrajectoryTracking_2015b_00/Nonlinear Transformation/Velocity Error /heave_error ==
  heave : Inport
  SwitchSchedule : Inport  Port=2
  Scope3 : Scope  NumInputPorts=2
  Sum5 : Sum  Inputs=|+-
  heave_d : Subsystem
  heave_err : Outport
  wires:
  heave/1 -> Scope3/1, Sum5/1
  Sum5/1 -> heave_err/1
  heave_d/1(heave_d) -> Scope3/2, Sum5/2
  SwitchSchedule/1 -> heave_d/1(SwitchSchedule)

== system TrajectoryTracking_2015b_00/Nonlinear Transformation/Velocity Error /pitch_error ==
  pitch : Inport
  SwitchSchedule : Inport  Port=2
  Scope3 : Scope  NumInputPorts=2
  Sum5 : Sum  Inputs=|+-
  pitch_d : Subsystem
  pitch_err : Outport
  wires:
  pitch/1 -> Scope3/1, Sum5/1
  Sum5/1 -> pitch_err/1
  SwitchSchedule/1 -> pitch_d/1(SwitchSchedule)
  pitch_d/1(pitch_d) -> Sum5/2, Scope3/2

== system TrajectoryTracking_2015b_00/Nonlinear Transformation/Velocity Error /roll_error ==
  roll : Inport
  SwitchSchedule : Inport  Port=2
  Scope3 : Scope  NumInputPorts=2
  Sum5 : Sum  Inputs=|+-
  roll_d : Subsystem
  roll_err : Outport
  wires:
  roll/1 -> Scope3/1, Sum5/1
  Sum5/1 -> roll_err/1
  SwitchSchedule/1 -> roll_d/1(SwitchSchedule)
  roll_d/1(roll_d) -> Scope3/2, Sum5/2

== system TrajectoryTracking_2015b_00/Nonlinear Transformation/Velocity Error /surge_error ==
  surge : Inport
  SwitchSchedule : Inport  Port=2
  Scope3 : Scope  NumInputPorts=2
  Sum5 : Sum  Inputs=|+-
  surge_d : Subsystem
  surge_err : Outport
  wires:
  surge/1 -> Scope3/1, Sum5/1
  Sum5/1 -> surge_err/1
  surge_d/1(surge_d) -> Scope3/2, Sum5/2
  SwitchSchedule/1 -> surge_d/1(SwitchSchedule)

== system TrajectoryTracking_2015b_00/Nonlinear Transformation/Velocity Error /sway_error ==
  sway : Inport
  SwitchSchedule : Inport  Port=2
  Scope3 : Scope  NumInputPorts=2
  Sum5 : Sum  Inputs=|+-
  sway_d : Subsystem
  sway_err : Outport
  wires:
  sway/1 -> Sum5/1
  Sum5/1 -> Scope3/1, sway_err/1
  SwitchSchedule/1 -> sway_d/1(SwitchSchedule)
  sway_d/1(sway_d) -> Scope3/2, Sum5/2

== system TrajectoryTracking_2015b_00/Nonlinear Transformation/Velocity Error /yaw_error ==
  pitch : Inport
  SwitchSchedule : Inport  Port=2
  Scope1 : Scope  NumInputPorts=2
  Scope3 : Scope  NumInputPorts=2
  Sum5 : Sum  Inputs=|+-
  yaw_d : Subsystem
  pitch_err : Outport
  wires:
  pitch/1 -> Scope1/1, Scope3/1, Sum5/1
  Sum5/1 -> pitch_err/1
  yaw_d/1(yaw_d) -> Sum5/2, Scope1/2, Scope3/2
  SwitchSchedule/1 -> yaw_d/1(SwitchSchedule)

== system TrajectoryTracking_2015b_00/Underwater Robot System/Underwater Robot System/DragCalculation ==
  nu : Inport
  Abs : Abs
  Constant : Constant  Value=veh.D
  Product : Product  Multiplication=Matrix(*)
  Product1 : Product
  HullDrag : Outport
  wires:
  Product/1 -> HullDrag/1
  Product1/1 -> Product/2
  Abs/1 -> Product1/1
  Constant/1 -> Product/1
  nu/1 -> Abs/1, Product1/2  "nu"

== system TrajectoryTracking_2015b_00/Underwater Robot System/Underwater Robot System/Dynamic2Kinematic(angular velocity) ==
  "p q r " : Inport
  Initial Integration Phi : Subsystem
  Initial Integration Value Generation Psi : Subsystem
  Initial Integration Value Generation Theta : Subsystem
  Mux1 : Mux  Inputs=3
  Rotation Angles to Direction Cosine Matrix : aerolibtransform2/Rotation Angles to Direction Cosine Matrix  rotationOrder=ZYX
  Selector : Selector  InputPortWidth=3  IndexOptions=Index vector (dialog)  Indices=[3 2 1]  OutputSizes=1
  phi theta psi : Integrator  InitialConditionSource=external
  phidot thetadot psidot1 : aerolib6dofsys/DCM & Euler Angles (Euler)/phidot thetadot psidot
  DCM : Outport
  Euler : Outport  Port=2
  Euler_dot : Outport  Port=3
  wires:
  Selector/1 -> Rotation Angles to Direction Cosine Matrix/1
  "p q r "/1 -> phidot thetadot psidot1/1
  phi theta psi/1 -> Selector/1, phidot thetadot psidot1/2, Euler/1
  phidot thetadot psidot1/1 -> Euler_dot/1, phi theta psi/1
  Rotation Angles to Direction Cosine Matrix/1 -> DCM/1
  Initial Integration Value Generation Psi/1(Initial Orientation Integration Value) -> Mux1/3
  Initial Integration Value Generation Theta/1(Initial Theta Integration Value) -> Mux1/2
  Mux1/1 -> phi theta psi/2
  Initial Integration Phi/1(Initial Phi Integration Value) -> Mux1/1

== system TrajectoryTracking_2015b_00/Underwater Robot System/Underwater Robot System/Initial Integration Value Generation Generalised Location ==
  Constant : Constant  Value=0
  Mux : Mux  Inputs=3
  Initial Location Integration Value : Outport
  wires:
  Constant/1 -> Mux/1, Mux/3, Mux/2
  Mux/1 -> Initial Location Integration Value/1

== system TrajectoryTracking_2015b_00/Underwater Robot System/Underwater Robot System/Underwater Robot Dynamics  ==
  tau_b : Inport
  6DOF Coriolis forces : Subsystem
  M_A : Constant  Value=veh.Ma
  M_RB : Constant  Value=veh.Mrb
  Product : Product  Inputs=/*  Multiplication=Matrix(*)  SaturateOnIntegerOverflow=on  OutDataTypeStr=Inherit: Same as first input
  Scope : Scope
  Selector1 : Selector  InputPortWidth=6  IndexOptions=Index vector (dialog)  Indices=[1 2 3]  OutputSizes=1
  Selector2 : Selector  InputPortWidth=6  IndexOptions=Index vector (dialog)  Indices=[4 5 6]  OutputSizes=1
  Sum : Sum  Inputs=|+-
  Sum2 : Sum  SaturateOnIntegerOverflow=on
  Velocity Integrator : Integrator
  v : Outport
  w_ib : Outport  Port=2
  wires:
  M_RB/1 -> Sum2/1
  M_A/1 -> Sum2/2
  Sum2/1 -> Product/1, 6DOF Coriolis forces/1(M)  "M"
  Selector2/1 -> w_ib/1  "w_nb"
  Product/1 -> Velocity Integrator/1  "(d/dt)nu"
  6DOF Coriolis forces/1(C(nu)nu) -> Sum/2, Scope/1
  Sum/1 -> Product/2
  Selector1/1 -> v/1  "v"
  Velocity Integrator/1 -> 6DOF Coriolis forces/2(nu), Selector2/1, Selector1/1  "nu"
  tau_b/1 -> Sum/1

== system TrajectoryTracking_2015b_00/Underwater Robot System/Underwater Robot System/transform to inertial world frame {i} ==
  v : Inport
  linear velocity transformation matrix : Inport  Port=2
  Product : Product  Multiplication=Matrix(*)  SaturateOnIntegerOverflow=on  InputSameDT=on  OutDataTypeStr=Inherit: Same as first input
  Reshape1 : Reshape  OutputDimensionality=Column vector (2-D)
  Reshape2 : Reshape
  Ve : Outport
  wires:
  Product/1 -> Reshape2/1
  Reshape1/1 -> Product/2
  v/1 -> Reshape1/1
  Reshape2/1 -> Ve/1
  linear velocity transformation matrix/1 -> Product/1

== system TrajectoryTracking_2015b_00/Nonlinear Transformation/Position Error /Nonlinear Orientation Transformation/Euler Angles to Angular Velocity Transfomration matrix ==
  theta : Inport
  Constant : Constant
  Constant1 : Constant  Value=0
  Mux : Mux  Inputs=9
  Reshape : Reshape  OutputDimensionality=Customize  OutputDimensions=[3,3]
  T21 : Fcn  Expr=sin(u(1))*tan(u(2))
  T22 : Fcn  Expr=cos(u(1))
  T23 : Fcn  Expr=sin(u(1))/cos(u(2))
  T31 : Fcn  Expr=cos(u(1))*tan(u(2))
  T32 : Fcn  Expr=-sin(u(1))
  T33 : Fcn  Expr=cos(u(1))/cos(u(2))
  T : Outport
  wires:
  Mux/1 -> Reshape/1
  Constant/1 -> Mux/1
  Constant1/1 -> Mux/2, Mux/3
  T21/1 -> Mux/4
  theta/1 -> T23/1, T33/1, T32/1, T31/1, T21/1, T22/1
  T22/1 -> Mux/5
  T23/1 -> Mux/6
  T31/1 -> Mux/7
  T32/1 -> Mux/8
  T33/1 -> Mux/9
  Reshape/1 -> T/1

== system TrajectoryTracking_2015b_00/Nonlinear Transformation/Position Error /Nonlinear Orientation Transformation/pitch_error ==
  pitch : Inport
  SwitchSchedule : Inport  Port=2
  Scope2 : Scope  NumInputPorts=2
  Sum13 : Sum  Inputs=|+-
  To Workspace : ToWorkspace  VariableName=theta_s  SaveFormat=Timeseries  SampleTime=-1
  theta_d : Subsystem
  pitch_err : Outport
  wires:
  pitch/1 -> To Workspace/1, Scope2/1, Sum13/1
  Sum13/1 -> pitch_err/1
  SwitchSchedule/1 -> theta_d/1(SwitchSchedule)
  theta_d/1(theta_d) -> Sum13/2, Scope2/2

== system TrajectoryTracking_2015b_00/Nonlinear Transformation/Position Error /Nonlinear Orientation Transformation/roll_error ==
  roll : Inport
  SwitchSchedule : Inport  Port=2
  Scope2 : Scope  NumInputPorts=2
  Sum13 : Sum  Inputs=|+-
  To Workspace : ToWorkspace  VariableName=phi_s  SaveFormat=Timeseries  SampleTime=-1
  phi_d : Subsystem
  roll_err : Outport
  wires:
  roll/1 -> To Workspace/1, Scope2/1, Sum13/1
  Sum13/1 -> roll_err/1
  SwitchSchedule/1 -> phi_d/1(SwitchSchedule)
  phi_d/1(phi_d) -> Scope2/2, Sum13/2

== system TrajectoryTracking_2015b_00/Nonlinear Transformation/Position Error /Nonlinear Orientation Transformation/yaw_error ==
  yaw : Inport
  SwitchSchedule : Inport  Port=2
  Scope2 : Scope  NumInputPorts=2
  Sum13 : Sum  Inputs=|+-
  To Workspace : ToWorkspace  VariableName=psi_s  SaveFormat=Timeseries  SampleTime=-1
  theta_d : Subsystem
  yaw_err : Outport
  wires:
  yaw/1 -> To Workspace/1, Scope2/1, Sum13/1
  Sum13/1 -> yaw_err/1
  theta_d/1(yaw_d) -> Scope2/2, Sum13/2
  SwitchSchedule/1 -> theta_d/1(SwitchSchedule)

== system TrajectoryTracking_2015b_00/Nonlinear Transformation/Position Error /Nonlinear Position Transformation/Euler Angles to inverse rotation matrix ==
  theta : Inport
  Mux : Mux  Inputs=2
  Mux1 : Mux  Inputs=9
  R11 : Fcn  Expr=u(5)*u(6)
  R12 : Fcn  Expr=u(5)*u(3)
  R13 : Fcn  Expr=-u(2)
  R21 : Fcn  Expr=-u(4)*u(3)+u(1)*u(2)*u(6)
  R22 : Fcn  Expr=u(4)*u(6)+u(1)*u(2)*u(3)
  R23 : Fcn  Expr=u(1)*u(5)
  R31 : Fcn  Expr=u(1)*u(3)+u(4)*u(2)*u(6)
  R32 : Fcn  Expr=-u(1)*u(6)+u(4)*u(2)*u(3)
  R33 : Fcn  Expr=u(4)*u(5)
  Reshape : Reshape  OutputDimensionality=Customize  OutputDimensions=[3,3]
  Trigonometric Function1 : Trigonometry  Operator=cos
  sin(theta) : Trigonometry
  inv(R) : Outport
  wires:
  theta/1 -> Trigonometric Function1/1, sin(theta)/1
  Trigonometric Function1/1 -> Mux/2
  sin(theta)/1 -> Mux/1
  Mux1/1 -> Reshape/1
  Mux/1 -> R32/1, R33/1, R23/1, R13/1, R22/1, R12/1, R31/1, R11/1, R21/1
  R11/1 -> Mux1/1
  R21/1 -> Mux1/2
  R31/1 -> Mux1/3
  R12/1 -> Mux1/4
  R22/1 -> Mux1/5
  R32/1 -> Mux1/6
  R13/1 -> Mux1/7
  R23/1 -> Mux1/8
  R33/1 -> Mux1/9
  Reshape/1 -> inv(R)/1

== system TrajectoryTracking_2015b_00/Nonlinear Transformation/Position Error /Nonlinear Position Transformation/x_error ==
  x : Inport
  SwitchSchedule : Inport  Port=2
  Scope2 : Scope  NumInputPorts=2
  Sum11 : Sum  Inputs=|+-
  To Workspace : ToWorkspace  VariableName=x_s  SaveFormat=Timeseries  SampleTime=-1
  To Workspace1 : ToWorkspace  VariableName=x_r  SaveFormat=Timeseries  SampleTime=-1
  x_d : Subsystem
  x_err : Outport
  wires:
  x/1 -> To Workspace/1, Scope2/1, Sum11/1
  Sum11/1 -> x_err/1
  SwitchSchedule/1 -> x_d/1(SwitchSchedule)
  x_d/1(x_d) -> Sum11/2, To Workspace1/1, Scope2/2

== system TrajectoryTracking_2015b_00/Nonlinear Transformation/Position Error /Nonlinear Position Transformation/y_error ==
  y : Inport
  SwitchSchedule : Inport  Port=2
  Scope2 : Scope  NumInputPorts=2
  Sum12 : Sum  Inputs=|+-
  To Workspace : ToWorkspace  VariableName=y_s  SaveFormat=Timeseries  SampleTime=-1
  To Workspace1 : ToWorkspace  VariableName=y_r  SaveFormat=Timeseries  SampleTime=-1
  y_d : Subsystem
  y_err : Outport
  wires:
  y/1 -> To Workspace/1, Scope2/1, Sum12/1
  Sum12/1 -> y_err/1
  SwitchSchedule/1 -> y_d/1(SwitchSchedule)
  y_d/1(y_d) -> To Workspace1/1, Sum12/2, Scope2/2

== system TrajectoryTracking_2015b_00/Nonlinear Transformation/Position Error /Nonlinear Position Transformation/z_error ==
  z : Inport
  SwitchSchedule : Inport  Port=2
  Scope2 : Scope  NumInputPorts=2
  Sum13 : Sum  Inputs=|+-
  To Workspace : ToWorkspace  VariableName=z_s  SaveFormat=Timeseries  SampleTime=-1
  To Workspace1 : ToWorkspace  VariableName=z_r  SaveFormat=Timeseries  SampleTime=-1
  z_d : Subsystem
  z_err : Outport
  wires:
  z/1 -> To Workspace/1, Scope2/1, Sum13/1
  Sum13/1 -> z_err/1
  SwitchSchedule/1 -> z_d/1(SwitchSchedule)
  z_d/1(z_d) -> To Workspace1/1, Scope2/2, Sum13/2

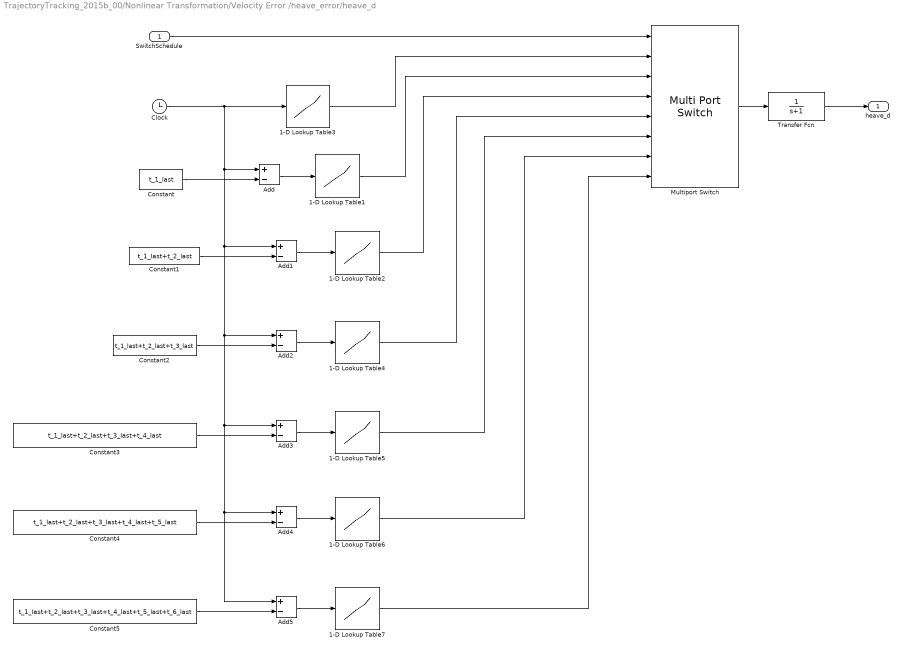
== system TrajectoryTracking_2015b_00/Nonlinear Transformation/Velocity Error /heave_error/heave_d ==
  SwitchSchedule : Inport
  1-D Lookup Table1 : Lookup_n-D  NumberOfTableDimensions=1  BreakpointsForDimension1=t_e_2  Table=linear_velocity_z_2  InternalRulePriority=Speed  RndMeth=Simplest  InputSameDT=on
  1-D Lookup Table2 : Lookup_n-D  NumberOfTableDimensions=1  BreakpointsForDimension1=t_e_3  Table=linear_velocity_z_3  InternalRulePriority=Speed  RndMeth=Simplest  InputSameDT=on
  1-D Lookup Table3 : Lookup_n-D  NumberOfTableDimensions=1  BreakpointsForDimension1=t_e_1  Table=linear_velocity_z_1  InternalRulePriority=Speed  RndMeth=Simplest  InputSameDT=on
  1-D Lookup Table4 : Lookup_n-D  NumberOfTableDimensions=1  BreakpointsForDimension1=t_e_4  Table=linear_velocity_z_4  InternalRulePriority=Speed  RndMeth=Simplest  InputSameDT=on
  1-D Lookup Table5 : Lookup_n-D  NumberOfTableDimensions=1  BreakpointsForDimension1=t_e_5  Table=linear_velocity_z_5  InternalRulePriority=Speed  RndMeth=Simplest  InputSameDT=on
  1-D Lookup Table6 : Lookup_n-D  NumberOfTableDimensions=1  BreakpointsForDimension1=t_e_6  Table=linear_velocity_z_6  InternalRulePriority=Speed  RndMeth=Simplest  InputSameDT=on
  1-D Lookup Table7 : Lookup_n-D  NumberOfTableDimensions=1  BreakpointsForDimension1=t_e_7  Table=linear_velocity_z_7  InternalRulePriority=Speed  RndMeth=Simplest  InputSameDT=on
  Add{,1..5} (6 alike) : Sum  Inputs=+-
  Clock : Clock
  Constant : Constant  Value=t_1_last
  Constant1 : Constant  Value=t_1_last+t_2_last
  Constant2 : Constant  Value=t_1_last+t_2_last+t_3_last
  Constant3 : Constant  Value=t_1_last+t_2_last+t_3_last+t_4_last
  Constant4 : Constant  Value=t_1_last+t_2_last+t_3_last+t_4_last+t_5_last
  Constant5 : Constant  Value=t_1_last+t_2_last+t_3_last+t_4_last+t_5_last+t_6_last
  Multiport Switch : MultiPortSwitch  Inputs=7
  Transfer Fcn : TransferFcn  Denominator=[1 1]
  heave_d : Outport
  wires:
  1-D Lookup Table1/1 -> Multiport Switch/3
  1-D Lookup Table3/1 -> Multiport Switch/2
  Constant/1 -> Add/2
  Multiport Switch/1 -> Transfer Fcn/1
  SwitchSchedule/1 -> Multiport Switch/1
  Add/1 -> 1-D Lookup Table1/1
  Constant1/1 -> Add1/2
  Add1/1 -> 1-D Lookup Table2/1
  1-D Lookup Table2/1 -> Multiport Switch/4
  Clock/1 -> Add5/1, Add4/1, Add3/1, Add2/1, Add1/1, Add/1, 1-D Lookup Table3/1
  Add2/1 -> 1-D Lookup Table4/1
  Constant2/1 -> Add2/2
  1-D Lookup Table4/1 -> Multiport Switch/5
  Transfer Fcn/1 -> heave_d/1
  Add3/1 -> 1-D Lookup Table5/1
  Constant3/1 -> Add3/2
  1-D Lookup Table5/1 -> Multiport Switch/6
  Add4/1 -> 1-D Lookup Table6/1
  Constant4/1 -> Add4/2
  1-D Lookup Table6/1 -> Multiport Switch/7
  Add5/1 -> 1-D Lookup Table7/1
  Constant5/1 -> Add5/2
  1-D Lookup Table7/1 -> Multiport Switch/8
